simulink model "wind_control"  (R2022b)
settings: Solver=VariableStepAuto  StartTime=0.0  StopTime=1800  RelTol=1e-3
values from neighbouring files (symbols this model uses):
  Cp = 0.48    [setup_wind_data.m]
  D = 220    [setup_wind_data.m]
  dt = mean(diff(t))    [setup_wind_data.m]
  Enom = battery_sizes(j)    [setup_wind_data.m]
  eta_c = 0.97    [setup_wind_data.m]
  eta_d = 0.97    [setup_wind_data.m]
  h = 0.05    [setup_wind_data.m]
  Ps_max = battery_sizes(j)    [setup_wind_data.m]
  Pw0 = 92 * P1_0    [setup_wind_data.m]
  Rdn_p = -ramp_constant * Csite / 60    (= -2)    [setup_wind_data.m]
  rho = 1.23    [setup_wind_data.m]
  Rup_p = ramp_constant * Csite / 60    (= 2)    [setup_wind_data.m]
  SOC0 = 0.5    [setup_wind_data.m]
  SOCmax = 0.8    [setup_wind_data.m]
  SOCmin = 0.2    [setup_wind_data.m]
  v_cin = 3    [setup_wind_data.m]
  v_coff = 25    [setup_wind_data.m]
undefined symbols (not defined in the file or in its folder): DiscIntNeverNeededParam
libraries: slpidlib x2, simulink x2
settings Model: Creator=efimlunev  LastModifiedBy=efimlunev

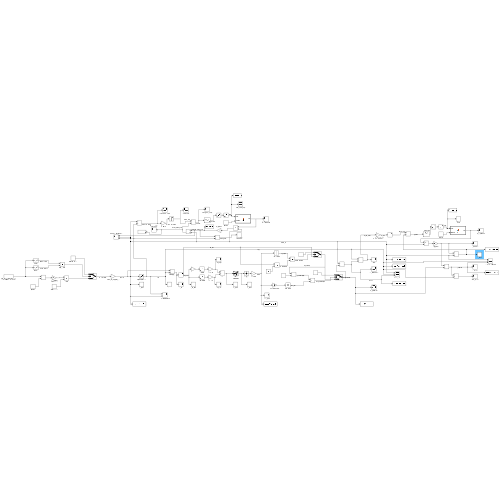
[thumbnail: Simulink's stored preview of the top-level diagram]
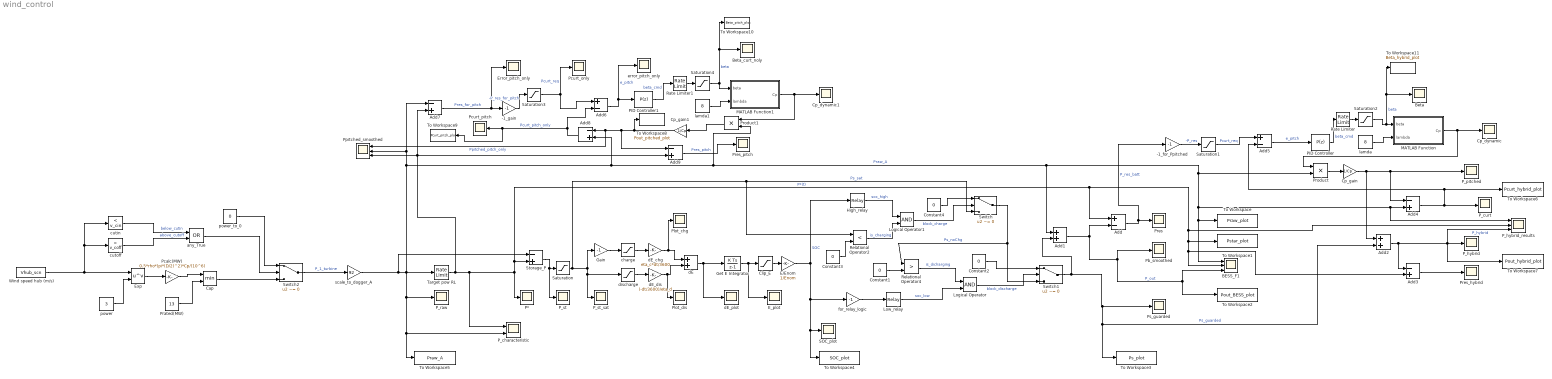
== system wind_control ==
  -1_for_Ppitched : Gain  Gain=-1
  -1_gain : Gain  Gain=-1
  Add : Sum  Inputs=+-
  Add1 : Sum
  Add2 : Sum
  Add{3..4,7..9} (5 alike) : Sum  Inputs=-+
  Add5 : Sum  Inputs=+-
  Add6 : Sum  Inputs=+-
  BESS_F1 : Scope  NumInputPorts=3
  Beta : Scope
  Beta_curt_noly : Scope
  Cap : MinMax  Inputs=2
  Clip_E : Saturate  UpperLimit=SOCmax*Enom  LowerLimit=SOCmin*Enom
  Constant{1..4} (4 alike) : Constant  Value=0
  Cp_dynamic : Scope
  Cp_dynamic1 : Scope
  Cp_gain : Gain  Gain=1/Cp
  Cp_gain1 : Gain  Gain=1/Cp
  E/Enom : Gain  Gain=1/Enom
  E_plot : Scope
  Error_pitch_only : Scope
  Exp : Math  Operator=pow
  Gain : Gain  Gain=-1
  Get E Integrator : DiscreteIntegrator  InitialCondition=SOC0*Enom  SampleTime=10  LimitOutput=on  UpperSaturationLimit=SOCmax*Enom  LowerSaturationLimit=SOCmin*Enom  ICPrevOutput=DiscIntNeverNeededParam  ICPrevScaledInput=DiscIntNeverNeededParam
  High_relay : Relay  OnSwitchValue=SOCmax  OffSwitchValue=SOCmax-h
  Logical Operator : Logic  AllPortsSameDT=off  OutDataTypeStr=boolean
  Logical Operator1 : Logic  AllPortsSameDT=off  OutDataTypeStr=boolean
  Low_relay : Relay  OnSwitchValue=-SOCmin  OffSwitchValue=-(SOCmin+h)
  MATLAB Function : MATLAB Function  TreatAsAtomicUnit=on
  MATLAB Function1 : MATLAB Function  TreatAsAtomicUnit=on
  P* : Scope
  PID Controller : slpidlib/PID Controller  Controller=P  Form=Parallel  TimeDomain=Discrete-time  UseExternalTs=off  SampleTime=10  IntegratorMethod=Forward Euler  FilterMethod=Forward Euler  ControllerParametersSource=internal  P=0.2  I=0.01  UseKiTs=off  D=0  N=100  UseFilter=on  TunerSelectOption=Transfer Function Based (PID Tuner App)  InitialConditionSource=internal  InitialConditionForIntegrator=0  InitialConditionForFilter=0  DifferentiatorICPrevScaledInput=0  ExternalReset=none  TrackingMode=off  Kt=1  LimitOutput=off  SatLimitsSource=internal  UpperSaturationLimit=inf  LowerSaturationLimit=-inf  LinearizeAsGain=on  AntiWindupMode=none  Kb=1  LimitIntegrator=off  UpperIntegratorSaturationLimit=inf  LowerIntegratorSaturationLimit=-inf  POutMin=[]  POutMax=[]  IOutMin=[]  IOutMax=[]  DOutMin=[]  DOutMax=[]  NOutMin=[]  NOutMax=[]  SumOutMin=[]  SumOutMax=[]  SaturationOutMin=[]  SaturationOutMax=[]  PParamMin=[]  PParamMax=[]  IParamMin=[]  IParamMax=[]  DParamMin=[]  DParamMax=[]  NParamMin=[]  NParamMax=[]  KbParamMin=[]  KbParamMax=[]  KtParamMin=[]  KtParamMax=[]  KbOutMin=[]  KbOutMax=[]  KtOutMin=[]  KtOutMax=[]  IntegratorOutMin=[]  IntegratorOutMax=[]  FilterOutMin=[]  FilterOutMax=[]  SumI1OutMin=[]  SumI1OutMax=[]  SumI2OutMin=[]  SumI2OutMax=[]  SumI3OutMin=[]  SumI3OutMax=[]  SumI4OutMin=[]  SumI4OutMax=[]  SumDOutMin=[]  SumDOutMax=[]  DifferentiatorOutMin=[]  DifferentiatorOutMax=[]  FilterDiffOutCoefMin=[]  FilterDiffOutCoefMax=[]  ReciprocalOutMin=[]  ReciprocalOutMax=[]  SumDenOutMin=[]  SumDenOutMax=[]  SumNumOutMin=[]  SumNumOutMax=[]  DivideOutMin=[]  DivideOutMax=[]  UdiffTsProdOutMin=[]  UdiffTsProdOutMax=[]  NTsProdOutMin=[]  NTsProdOutMax=[]  UintegralTsProdOutMin=[]  UintegralTsProdOutMax=[]  UngainTsProdOutMin=[]  UngainTsProdOutMax=[]  ClampingZeroOutDataTypeStr=Inherit: Inherit via back propagation  ClampingZeroOutMin=[]  ClampingZeroOutMax=[]  FilterDenConstantOutDataTypeStr=Inherit: Inherit via back propagation  FilterDenConstantOutMin=[]  FilterDenConstantOutMax=[]  PCopyOutDataTypeStr=Inherit: Inherit via back propagation  PCopyOutMin=[]  PCopyOutMax=[]  NCopyOutDataTypeStr=Inherit: Inherit via back propagation  NCopyOutMin=[]  NCopyOutMax=[]  IntegratorContinuousStateAttributes=''  IntegratorStateMustResolveToSignalObject=off  IntegratorRTWStateStorageClass=Auto  FilterContinuousStateAttributes=''  FilterStateMustResolveToSignalObject=off  FilterRTWStateStorageClass=Auto  ParallelPVariant=InternalParameters  IdealPVariant=Disabled  IVariant=Disabled  DVariant=Disabled  IntegratorVariant=Disabled  SatVariant=Disabled  AWVariant=Disabled  PCopyVariant=Disabled  TRVariant=Disabled  FdbkBlocksVariant=Forward  IdealPFdbkVariant=Disabled  SatFdbkVariant=Disabled  DerivativeFilterVariant=Disabled  NVariant=Disabled  NCopyVariant=Disabled_SignalSpec  FilterICVariant=Disabled  IntegratorICVariant=Disabled  ExternalResetVariant=Disabled  TRSumVariant=Passthrough  SumFdbkVariant=Disabled  SumVariant=Passthrough_P  TsampFilterVariant=InternalTs  TsampNgainVariant=Passthrough  TsampIntegralVariant=Disabled_SignalSpec  ExternalSaturationOutDataTypeStr=Inherit: Same as second input
  PID Controller1 : slpidlib/PID Controller  Controller=P  Form=Parallel  TimeDomain=Discrete-time  UseExternalTs=off  SampleTime=10  IntegratorMethod=Forward Euler  FilterMethod=Forward Euler  ControllerParametersSource=internal  P=0.2  I=0.01  UseKiTs=off  D=0  N=100  UseFilter=on  TunerSelectOption=Transfer Function Based (PID Tuner App)  InitialConditionSource=internal  InitialConditionForIntegrator=0  InitialConditionForFilter=0  DifferentiatorICPrevScaledInput=0  ExternalReset=none  TrackingMode=off  Kt=1  LimitOutput=off  SatLimitsSource=internal  UpperSaturationLimit=inf  LowerSaturationLimit=-inf  LinearizeAsGain=on  AntiWindupMode=none  Kb=1  LimitIntegrator=off  UpperIntegratorSaturationLimit=inf  LowerIntegratorSaturationLimit=-inf  POutMin=[]  POutMax=[]  IOutMin=[]  IOutMax=[]  DOutMin=[]  DOutMax=[]  NOutMin=[]  NOutMax=[]  SumOutMin=[]  SumOutMax=[]  SaturationOutMin=[]  SaturationOutMax=[]  PParamMin=[]  PParamMax=[]  IParamMin=[]  IParamMax=[]  DParamMin=[]  DParamMax=[]  NParamMin=[]  NParamMax=[]  KbParamMin=[]  KbParamMax=[]  KtParamMin=[]  KtParamMax=[]  KbOutMin=[]  KbOutMax=[]  KtOutMin=[]  KtOutMax=[]  IntegratorOutMin=[]  IntegratorOutMax=[]  FilterOutMin=[]  FilterOutMax=[]  SumI1OutMin=[]  SumI1OutMax=[]  SumI2OutMin=[]  SumI2OutMax=[]  SumI3OutMin=[]  SumI3OutMax=[]  SumI4OutMin=[]  SumI4OutMax=[]  SumDOutMin=[]  SumDOutMax=[]  DifferentiatorOutMin=[]  DifferentiatorOutMax=[]  FilterDiffOutCoefMin=[]  FilterDiffOutCoefMax=[]  ReciprocalOutMin=[]  ReciprocalOutMax=[]  SumDenOutMin=[]  SumDenOutMax=[]  SumNumOutMin=[]  SumNumOutMax=[]  DivideOutMin=[]  DivideOutMax=[]  UdiffTsProdOutMin=[]  UdiffTsProdOutMax=[]  NTsProdOutMin=[]  NTsProdOutMax=[]  UintegralTsProdOutMin=[]  UintegralTsProdOutMax=[]  UngainTsProdOutMin=[]  UngainTsProdOutMax=[]  ClampingZeroOutDataTypeStr=Inherit: Inherit via back propagation  ClampingZeroOutMin=[]  ClampingZeroOutMax=[]  FilterDenConstantOutDataTypeStr=Inherit: Inherit via back propagation  FilterDenConstantOutMin=[]  FilterDenConstantOutMax=[]  PCopyOutDataTypeStr=Inherit: Inherit via back propagation  PCopyOutMin=[]  PCopyOutMax=[]  NCopyOutDataTypeStr=Inherit: Inherit via back propagation  NCopyOutMin=[]  NCopyOutMax=[]  IntegratorContinuousStateAttributes=''  IntegratorStateMustResolveToSignalObject=off  IntegratorRTWStateStorageClass=Auto  FilterContinuousStateAttributes=''  FilterStateMustResolveToSignalObject=off  FilterRTWStateStorageClass=Auto  ParallelPVariant=InternalParameters  IdealPVariant=Disabled  IVariant=Disabled  DVariant=Disabled  IntegratorVariant=Disabled  SatVariant=Disabled  AWVariant=Disabled  PCopyVariant=Disabled  TRVariant=Disabled  FdbkBlocksVariant=Forward  IdealPFdbkVariant=Disabled  SatFdbkVariant=Disabled  DerivativeFilterVariant=Disabled  NVariant=Disabled  NCopyVariant=Disabled_SignalSpec  FilterICVariant=Disabled  IntegratorICVariant=Disabled  ExternalResetVariant=Disabled  TRSumVariant=Passthrough  SumFdbkVariant=Disabled  SumVariant=Passthrough_P  TsampFilterVariant=InternalTs  TsampNgainVariant=Passthrough  TsampIntegralVariant=Disabled_SignalSpec  ExternalSaturationOutDataTypeStr=Inherit: Same as second input
  P_characteristic : Scope  NumInputPorts=2
  P_curt : Scope
  P_hybrid : Scope
  P_hybrid_results : Scope  NumInputPorts=3
  P_pitched : Scope
  P_raw : Scope
  P_st : Scope
  P_st_sat : Scope
  Pb_smoothed : Scope
  Pcalc(MW) : Gain  Gain=0.5*rho*(pi*(D/2)^2)*Cp/(10^6)
  Pcurt_only : Scope
  Pcurt_pitch : Scope
  Plot_chg : Scope
  Plot_dis : Scope
  Ppitched_smoothed : Scope  NumInputPorts=3
  Prated(MW) : Constant  Value=13
  Pres : Scope
  Pres_hybrid : Scope
  Pres_pitch : Scope
  Product : Product
  Product1 : Product
  Ps_guarded : Scope
  Rate Limiter : RateLimiter  RisingSlewLimit=8  FallingSlewLimit=-8  SampleTimeMode=inherited
  Rate Limiter1 : RateLimiter  RisingSlewLimit=8  FallingSlewLimit=-8  SampleTimeMode=inherited
  Relational Operator2 : RelationalOperator  Operator=<  OutDataTypeStr=boolean  RndMeth=Simplest  InputSameDT=off
  Relational Operator4 : RelationalOperator  Operator=>  OutDataTypeStr=boolean  RndMeth=Simplest  InputSameDT=off
  SOC_plot : Scope
  Saturation : Saturate  UpperLimit=Ps_max  LowerLimit=-Ps_max
  Saturation1 : Saturate  UpperLimit=inf  LowerLimit=0
  Saturation2 : Saturate  UpperLimit=25  LowerLimit=0
  Saturation3 : Saturate  UpperLimit=inf  LowerLimit=0
  Saturation4 : Saturate  UpperLimit=25  LowerLimit=0
  Storage_P : Sum  Inputs=-+
  Switch : Switch  Criteria=u2 ~= 0  SaturateOnIntegerOverflow=off  InputSameDT=off
  Switch1 : Switch  Criteria=u2 ~= 0  SaturateOnIntegerOverflow=off  InputSameDT=off
  Switch2 : Switch  Criteria=u2 ~= 0  SaturateOnIntegerOverflow=off  InputSameDT=off
  Target pow RL : RateLimiter  RisingSlewLimit=Rup_p  FallingSlewLimit=Rdn_p  SampleTimeMode=inherited  InitialCondition=Pw0
  To Workspace : ToWorkspace  VariableName=Praw_plot  SampleTime=-1
  To Workspace1 : ToWorkspace  VariableName=Pstar_plot  SampleTime=-1
  To Workspace10 : ToWorkspace  VariableName=Beta_pitch_plot  SampleTime=-1
  To Workspace11 : ToWorkspace  VariableName=Beta_hybrid_plot  SampleTime=-1
  To Workspace2 : ToWorkspace  VariableName=Pout_BESS_plot  SampleTime=-1
  To Workspace3 : ToWorkspace  VariableName=Ps_plot  SampleTime=-1
  To Workspace4 : ToWorkspace  VariableName=SOC_plot  SampleTime=-1
  To Workspace5 : ToWorkspace  VariableName=Praw_A  SampleTime=-1
  To Workspace6 : ToWorkspace  VariableName=Pcurt_hybrid_plot  SampleTime=-1
  To Workspace7 : ToWorkspace  VariableName=Pout_hybrid_plot  SampleTime=-1
  To Workspace8 : ToWorkspace  VariableName=Pout_pitched_plot  SampleTime=-1
  To Workspace9 : ToWorkspace  VariableName=Pcurt_pitch_plot  SampleTime=-1
  Wind speed hub (m/s) : FromWorkspace  VariableName=Vhub_scn  SampleTime=10
  any_True : Logic  Operator=OR  AllPortsSameDT=off  OutDataTypeStr=boolean
  charge : Saturate  UpperLimit=Inf  LowerLimit=0
  cutin : simulink/Logic and Bit Operations/Compare To Constant  relop=<  const=v_cin  OutDataTypeStr=boolean
  cutoff : simulink/Logic and Bit Operations/Compare To Constant  relop=>  const=v_coff  OutDataTypeStr=boolean
  dE : Sum
  dE_chg : Gain  Gain=eta_c*dt/3600
  dE_dis : Gain  Gain=(-dt/3600)/eta_d
  dE_plot : Scope
  discharge : Saturate  UpperLimit=Inf  LowerLimit=0
  error_pitch_only : Scope
  for_relay_logic : Gain  Gain=-1
  lamda : Constant  Value=8
  lamda1 : Constant  Value=8
  power : Constant  Value=3
  power_to_0 : Constant  Value=0
  scale_to_dogger_A : Gain  Gain=92
  wires:
  Target pow RL/1 -> P_characteristic/1, P_hybrid_results/2, Add3/2, BESS_F1/2, To Workspace1/1, Add/1, Storage_P/2, P*/1, Ppitched_smoothed/3, Add9/2, Add7/2  "P*(t)"
  Storage_P/1 -> Saturation/1, P_st/1
  Saturation/1 -> Relational Operator2/1, Switch/3, P_st_sat/1, discharge/1, Gain/1  "Ps_sat"
  Gain/1 -> charge/1
  dE_dis/1 -> Plot_dis/1, dE/2
  dE_chg/1 -> Plot_chg/1, dE/1
  dE/1 -> dE_plot/1, Get E Integrator/1
  Get E Integrator/1 -> Clip_E/1, E_plot/1
  discharge/1 -> dE_dis/1
  charge/1 -> dE_chg/1
  E/Enom/1 -> High_relay/1, for_relay_logic/1, To Workspace4/1, SOC_plot/1  "SOC"
  High_relay/1 -> Logical Operator1/1  "soc_high"
  Constant3/1 -> Relational Operator2/2
  Relational Operator2/1 -> Logical Operator1/2  "is_charging"
  Switch/1 -> Relational Operator4/1, Switch1/3  "Ps_noChg"
  Constant1/1 -> Relational Operator4/2
  Relational Operator4/1 -> Logical Operator/1  "is_dicharging"
  Low_relay/1 -> Logical Operator/2  "soc_low"
  Switch1/1 -> Add1/2, Add2/2, To Workspace3/1, Ps_guarded/1  "Ps_guarded"
  Clip_E/1 -> E/Enom/1
  Logical Operator1/1 -> Switch/2  "block_charge"
  Constant4/1 -> Switch/1
  Constant2/1 -> Switch1/1
  Logical Operator/1 -> Switch1/2  "block_discharge"
  Wind speed hub (m/s)/1 -> cutin/1, cutoff/1, Exp/1
  power/1 -> Exp/2
  Exp/1 -> Pcalc(MW)/1
  Pcalc(MW)/1 -> Cap/1
  Prated(MW)/1 -> Cap/2
  cutoff/1 -> any_True/2  "above_cutoff"
  cutin/1 -> any_True/1  "below_cutin"
  any_True/1 -> Switch2/2
  power_to_0/1 -> Switch2/1
  Cap/1 -> Switch2/3
  scale_to_dogger_A/1 -> Target pow RL/1, Ppitched_smoothed/2, Add7/1, Product1/2, Add1/1, BESS_F1/1, To Workspace/1, P_hybrid_results/1, Add4/2, Product/2, Add8/2, P_characteristic/2, To Workspace5/1, P_raw/1, Storage_P/1  "Praw_A"
  Switch2/1 -> scale_to_dogger_A/1  "P_1_turbine"
  for_relay_logic/1 -> Low_relay/1
  Add1/1 -> Add/2, BESS_F1/3, To Workspace2/1, Pb_smoothed/1  "P_out"
  Add/1 -> Pres/1, -1_for_Ppitched/1  "P_res_batt"
  -1_for_Ppitched/1 -> Saturation1/1  "-P_res"
  Saturation1/1 -> Add5/1  "Pcurt_req"
  PID Controller/1 -> Rate Limiter/1  "beta_cmd"
  Rate Limiter/1 -> Saturation2/1
  Saturation2/1 -> Beta/1, To Workspace11/1, MATLAB Function/1(beta)  "beta"
  lamda/1 -> MATLAB Function/2(lambda)
  MATLAB Function/1(Cp) -> Product/1, Cp_dynamic/1
  Add2/1 -> To Workspace7/1, P_hybrid_results/3, P_hybrid/1, Add3/1  "P_hybrid"
  Add3/1 -> Pres_hybrid/1
  Product/1 -> Cp_gain/1
  Cp_gain/1 -> P_pitched/1, Add4/1, Add2/1
  Add5/1 -> PID Controller/1  "e_pitch"
  Add4/1 -> Add5/2, To Workspace6/1, P_curt/1
  lamda1/1 -> MATLAB Function1/2(lambda)
  PID Controller1/1 -> Rate Limiter1/1  "beta_cmd"
  MATLAB Function1/1(Cp) -> Product1/1, Cp_dynamic1/1
  Saturation3/1 -> Add6/1, Pcurt_only/1  "Pcurt_req"
  Saturation4/1 -> To Workspace10/1, Beta_curt_noly/1, MATLAB Function1/1(beta)  "beta"
  Rate Limiter1/1 -> Saturation4/1
  -1_gain/1 -> Saturation3/1  "-P_res_for_pitch"
  Product1/1 -> Cp_gain1/1
  Add7/1 -> Error_pitch_only/1, -1_gain/1  "Pres_for_pitch"
  Add6/1 -> error_pitch_only/1, PID Controller1/1  "e_pitch"
  Cp_gain1/1 -> To Workspace8/1, Add9/1, Ppitched_smoothed/1, Add8/1  "Ppitched_pitch_only"
  Add8/1 -> To Workspace9/1, Pcurt_pitch/1, Add6/2  "Pcurt_pitch_only"
  Add9/1 -> Pres_pitch/1  "Pres_pitch"

== matlab function wind_control/MATLAB Function ==
  data: beta input; Cp output; lambda input
function Cp = fcn(beta, lambda)
% beta in degrees
% lambda assumed constant, e.g. 8

c1 = 0.5176;
c2 = 116;
c3 = 0.4;
c4 = 5;
c5 = 21;
c6 = 0.0068;

inv_lambda_i = 1/(lambda + 0.08*beta) - 0.035/(beta^3 + 1);

if inv_lambda_i <= 0
    Cp = 0;
    return
end

lambda_i = 1/inv_lambda_i;

Cp = c1 * (116/lambda_i - 0.4*beta - 5) * exp(-21/lambda_i) + 0.0068*lambda;

% physical bounds
Cp = max(0, min(Cp, 0.5));

== matlab function wind_control/MATLAB Function1 ==
  data: beta input; Cp output; lambda input
function Cp = fcn(beta, lambda)
% beta in degrees
% lambda assumed constant, e.g. 8

c1 = 0.5176;
c2 = 116;
c3 = 0.4;
c4 = 5;
c5 = 21;
c6 = 0.0068;

inv_lambda_i = 1/(lambda + 0.08*beta) - 0.035/(beta^3 + 1);

if inv_lambda_i <= 0
    Cp = 0;
    return
end

lambda_i = 1/inv_lambda_i;

Cp = c1 * (116/lambda_i - 0.4*beta - 5) * exp(-21/lambda_i) + 0.0068*lambda;

% physical bounds
Cp = max(0, min(Cp, 0.5));
